simulink model "Model_InterpretationEngine64"  (R2022b)
settings: Solver=FixedStepDiscrete  StartTime=0.0  StopTime=5  RelTol=1e-3  EnableMultiTasking=on
InitFcn:
  | % Initialize model
  | ModelSettings=BTConfig.GetModelSettings();
  | 
  | ModelSettings.Validate();
  | 
  | ModelInit;
  | 
  | 
  | % load library data
  | GainLibrary_data;
  | % Load saved values from partition process
  | CapturedConstMask.LoadMapFromFile(bdroot)
  | % Load saved values from partition process
  | TSP_Mask.LoadMapFromFile(bdroot)
StartFcn:
  | % make sure all the simulated RTC requests are found
  | %RTC_SIM_OBJ.ValidateREQs();
undefined symbols (not defined in the file or in its folder): NumHFRefBPF, NumHFRefLPF
libraries: StateVar x112, TSP x56, FeaturePath x24
(part 1 of 5)
settings Model: Creator=kl13806  LastModifiedBy=mp55777
settings DataIOCC: ReturnWorkspaceOutputs=off
settings OptimizationCC: DefaultParameterBehavior=Inlined  DefaultUnderspecifiedDataType=single  EfficientTunableParamExpr=on
settings DebuggingCC: MergeDetectMultiDrivingBlocksExec=none  InheritedTsInSrcMsg=none  MultiTaskDSMMsg=none  ParameterPrecisionLossMsg=none  ParameterTunabilityLossMsg=error  UnconnectedInputMsg=warning  UnconnectedOutputMsg=warning  UnconnectedLineMsg=warning  UnknownTsInhSupMsg=none  SFUnexpectedBacktrackingDiag=warning  SFNoUnconditionalDefaultTransitionDiag=warning  SFExecutionAtInitializationDiag=none  SFMachineParentedDataDiag=warning
settings HardwareCC: ProdBitPerPointer=32  ProdBitPerSizeT=32  ProdBitPerPtrDiffT=32  ProdWordSize=32  ProdHWDeviceType=Intel->x86-32 (Windows32)  TargetBitPerPointer=64  TargetBitPerSizeT=64  TargetBitPerPtrDiffT=64  TargetLongLongMode=on  TargetIntDivRoundTo=Zero  TargetEndianess=LittleEndian  TargetWordSize=64  TargetHWDeviceType=MATLAB Host  ProdEqTarget=off
settings ModelReferenceCC: EnableRefExpFcnMdlSchedulingChecks=on  ModelReferenceNumInstancesAllowed=Single
settings SFSimCC: MATLABDynamicMemAlloc=off
settings RTWCC: Description=Embedded Coder (host-based shared library target)  SystemTargetFile=ert_shrlib.tlc  TLCOptions="-aTALARIA_ENGINE=\"Interpretation\""  TemplateMakefile=ert_default_tmf  RTWVerbose=off  RetainRTWFile=on  Toolchain=MinGW64 | gmake (64-bit Windows)  IncludeHyperlinkInReport=on
settings RTWCC: CustomHeaderCode=|
  | // Auto-generated code for model Model
  | /**** TSP TOKEN COMPATIBILITY HASH VALUES ****/
  | #define TSP_COMPAT {0xD202EF8DUL, 0xD716E441UL, 0xBB1AC2DBUL, 0x70247352UL, 0xD202EF8DUL}
  | #define TSP_COMPAT_NAME {"InputSelect", "PreAmp", "Near", "PostProcess", "TestRouter"}
  | #define TSP_COMPAT_NAME_HASH {0xF8044409UL, 0xC3A89EEBUL, 0xD67EB32FUL, 0x062DAD3BUL, 0x8CC5BE54UL}
  | /**** COMPAT HASH VALUES BY MODULE ****/
  | #define INPUTSELECT_TSP_COMPAT 0xD202EF8DUL
  | #define PREAMP_TSP_COMPAT 0xD716E441UL
  | #define NEAR_TSP_COMPAT 0xBB1AC2DBUL
  | #define POSTPROCESS_TSP_COMPAT 0x70247352UL
  | #define TESTROUTER_TSP_COMPAT 0xD202EF8DUL
  | /**** NAME HASH VALUES BY MODULE ****/
  | #define INPUTSELECT_TSP_NAME_HASH 0xF8044409UL
  | #define PREAMP_TSP_NAME_HASH 0xC3A89EEBUL
  | #define NEAR_TSP_NAME_HASH 0xD67EB32FUL
  | #define POSTPROCESS_TSP_NAME_HASH 0x062DAD3BUL
  | #define TESTROUTER_TSP_NAME_HASH 0x8CC5BE54UL
settings CodeAppCC: ForceParamTrailComments=on  IgnoreCustomStorageClasses=off  MaxIdLength=128  OperatorAnnotations=on  SimulinkDataObjDesc=on  SFDataObjDesc=on  MATLABFcnDesc=on  InsertBlockDesc=on  StateflowObjectComments=on  MATLABSourceComments=on
settings STFCustomTargetCC: TargetLangStandard=C99 (ISO)  MultiwordLength=256  ParMdlRefBuildCompliant=on  CompOptLevelCompliant=on  CombineOutputUpdateFcns=on  ERTCustomFileBanners=on  SupportContinuousTime=off  SupportNonInlinedSFcns=off  RemoveResetFunc=on  SupportVariableSizeSignals=on  MATLABClassNameForMDSCustomization=Simulink.SoftwareTarget.ERTCustomization  ModelStepFunctionPrototypeControlCompliant=on  UseToolchainInfoCompliant=on  SystemTargetFile=ert_shrlib.tlc
settings ERTTargetCC: TargetLangStandard=C99 (ISO)  ConcurrentExecutionCompliant=off  SupportVariableSizeSignals=on  CPPClassGenCompliant=off  InlinedParameterPlacement=NonHierarchical  ERTCustomFileTemplate=interpretation_dll.tlc  IndentStyle=Allman  IndentSize=4

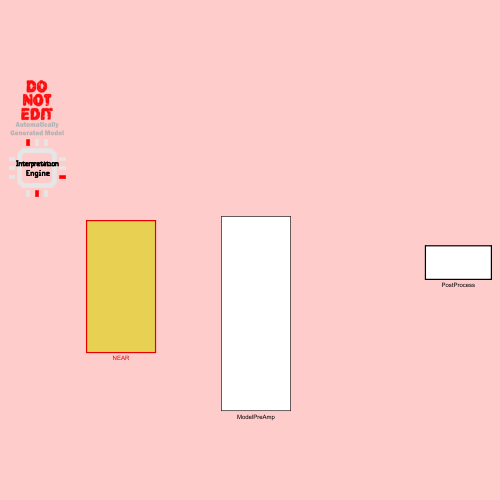
[thumbnail: Simulink's stored preview of the top-level diagram]
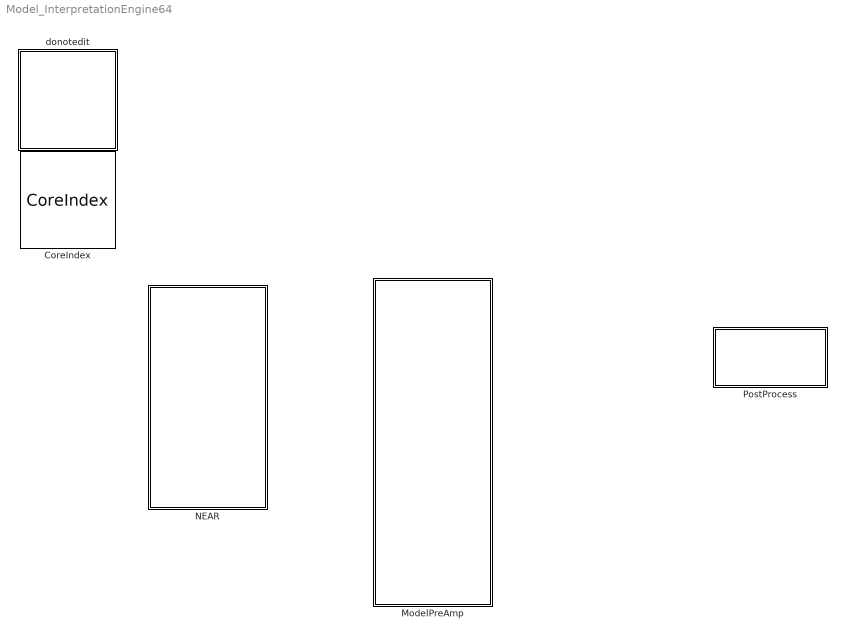
== system Model_InterpretationEngine64 ==
  CoreIndex : FeaturePath/CoreIndex  Role=Interpretation Engine  CoreIndex=10  Config=[]  AddressingMode=Indirect core determination via table lookup (i.e. use Partition blocks)  CrossCoreApi=None  CrossCoreAllocation=None  CrossCoreSampleTime=-1  BasePeriod=[]  TriggerInit=[440 234 535 331]
      settings: SourceProductName=Bose Talaria
  ModelPreAmp : Subsystem  mask{Config=ModelSettings.ModelPreAmp}
      mask prompts: Config "PreAmpConfig"
  NEAR : Subsystem  TreatAsAtomicUnit=on  mask{Config=ModelSettings.NearConfig}
      mask prompts: Config "NearConfig"
  PostProcess : Subsystem  TreatAsAtomicUnit=on  mask{Config=ModelSettings.PostProcess}
      mask prompts: Config "PostProcessConfig"
  donotedit : Subsystem
      settings: OpenFcn=Model
      mask Display: image('DoNotEdit.svg');

== system Model_InterpretationEngine64/ModelPreAmp ==
  DecRate : Subsystem
  FeaturePath : FeaturePath/FeaturePath  FeatureName=PreAmp  IsGroup=on  GroupNumber=2  IsModule=on  TriggerInit=[-135 -246 -20 -139]
      settings: SourceProductName=Bose Talaria

== system Model_InterpretationEngine64/NEAR ==
  FeaturePath : FeaturePath/FeaturePath  FeatureName=Near  IsGroup=on  GroupNumber=1  IsModule=on  TriggerInit=[15 -306 130 -199]
      settings: SourceProductName=Bose Talaria
  Near1p1 : Subsystem  mask{Config=Config.Near}
      mask prompts: Config "Near1p1Config"
      mask init:
      | blkh=gcbh;
      | Config=BTConfig.Assert(blkh,Config);
      | % sample_rate_in_hertz                        = near.sample_rate_in_hertz;
      | % frame_size                                  = near.frame_size;
      | % ann_sysin_channel_count                     = near.ann_sysin_channel_count;
      | % front_peripheral_channel_count              = near.front_peripheral_channel_count;
      | % NEAR1p1FrontPeripheralChannelCountFullRate  = near.NEAR1p1FrontPeripheralChannelCountFullRate;
      | % NearWbAnnCount                              = near.NearWbAnnCount;
      | % headrest_count                              = near.headrest_count;
      | % channels_per_headrest                       = near.channels_per_headrest;
      | % decimation_factor                           = near.decimation_factor;
      | % rear_channel_count                          = near.rear_channel_count;
      | % vm                                          = near.vm;
      | % decimated_frame_size                        = near.decimated_frame_size;
      | % decimated_sample_rate_in_hertz              = near.decimated_sample_rate_in_hertz;
      | Config.Validate();
      | Config.DoMaskInit(blkh);

== system Model_InterpretationEngine64/PostProcess ==
  FeaturePath : FeaturePath/FeaturePath  FeatureName=PostProcess  IsGroup=on  GroupNumber=3  IsModule=on  TriggerInit=[85 -186 200 -79]
      settings: SourceProductName=Bose Talaria
  PostProcess : Subsystem  TreatAsAtomicUnit=on
      settings: RTWSystemCode=Nonreusable function  RTWFcnNameOpts=Use subsystem name  RTWFileNameOpts=Use subsystem name  FunctionWithSeparateData=on

== system Model_InterpretationEngine64/donotedit ==

== system Model_InterpretationEngine64/ModelPreAmp/DecRate ==
  AudioPilot35 : Subsystem  TreatAsAtomicUnit=on
      settings: RTWFcnNameOpts=Use subsystem name  RTWFileNameOpts=Use subsystem name  FunctionWithSeparateData=on
  Medusa5H1 : Subsystem

== system Model_InterpretationEngine64/NEAR/Near1p1 ==
  VolumeMute : Subsystem  mask{Config=Config.VolumeMute}
      mask prompts: Config "VolumeMuteConfig"
      mask init:
      | blkh=gcbh;
      | Config=BTConfig.Assert(blkh,Config);
      | 
      | Config.Validate();
      | Config.DoMaskInit(blkh);

== system Model_InterpretationEngine64/PostProcess/PostProcess ==
  EnergyLimiter : Subsystem

== system Model_InterpretationEngine64/ModelPreAmp/DecRate/AudioPilot35 ==
  Audiopilot_3_5 : Subsystem  mask(AudioPilot 3.5){FeatureName=Audiopilot, InputAudioMode=Stereo - 2 Channels, NoiseEstimationMode=Regular, IncludeSpumTails=off, IncludeIgnoreMicFlag=off, Config=Config.Audiopilot}
      mask prompts: FeatureName "Feature Name:"; InputAudioMode "Input Audio Mode"; NoiseEstimationMode "Mode"; IncludeSpumTails "Include SPUM Tails as Reference Channels for High-Frequency Noise Estimator"; IncludeIgnoreMicFlag "Include Ignore Microphone Flag as Input"; Config "Audiopilot_3_5Config"
      mask help:
      | This is the top level model implementing AudioPilot 3.5.
      | It is configurable to accommodate both stereo inputs and surround inputs.  It can also reconfigure itself to become a speed-only implementation. For the regular implementation, there are two options. One is to allow a flag signal to instruct the algorithm to ignore the microphone signal; the other is to include in the set of "high-passed" reference channels the 2 channels representing the SPUM tails from the Medusa Upmixer.
      | Build Time Configuration settings typically set for this block include the frame size and the sample rate of the input audio. Other options include the type of code generation and whether all RTC blocks will generate a response.
      mask init:
      | blkh = gcbh;
      | 
      | Config = BTConfig.Assert(blkh,Config);
      | Config.Validate();
      | 
      | FrameSize = Config.FrameSize;
      | SampleRate = Config.SampleRateHz;
      |  
      | % Make the choice for the Noise Estimation Variant
      | Audiopilot_3_5Mask.ConfigureVariant(blkh,NoiseEstimationMode);
      | 
      | % Set up the number of audio channels for each input
      | [NumMicChannels,NumMusicChannels, ...
      |     NumHFRefLPF,NumHFRefBPF,NumLFRef] = ...
      |     Audiopilot_3_5Mask.ChannelSetUp(blkh,InputAudioMode,...
      |                 NoiseEstimationMode,IncludeSpumTails);
      | 
      | % Configure RTC responses            
      | Audiopilot_3_5Mask.ConfigureRtcResponses(blkh,...
      |                 Config.EnableRtcResponse)           
      | 
      | % Configure the Model according to Mask Parameters   
      | Audiopilot_3_5Mask.ConfigureModel(blkh,InputAudioMode,...
      |     NoiseEstimationMode,IncludeIgnoreMicFlag);
      | 
      | BTConfig.InitSetFeatureIfPresent(blkh,'FeatureName');
      mask TypeOptions FeatureName: FeaturePath/FeatureName
      mask TypeOptions InputAudioMode: Stereo - 2 Channels | Surround - 6 Channels
      mask TypeOptions NoiseEstimationMode: Regular | Speed Only
      mask Callback NoiseEstimationMode: Audiopilot_3_5Mask.NoiseEstimationModeCallBack(gcbh);
      mask Callback Config: BTConfig.CallbackHideIfPresent(gcbh,{'FeatureName'});
      mask DialogControl DTCTitle Prompt: <b> Design Time Configuration </b>
      mask DialogControl NoiseEstimationBox Prompt: Noise Estimation
      mask DialogControl BTCTitle Prompt: <b> Build Time Configuration </b>
  EntertainmentLevelDetection : Subsystem  mask(Level Detector for AudioPilot, Dyanmic EQ, Fan and Boost-on-Demand){NumInputChannels=Config.AudiopilotNumMusicIn, FANEnable=off, BODEnable=off, Config=Config.LDCfg}
      mask prompts: NumInputChannels "Number of Input Channels"; FANEnable "FAN (amplifier fan control)"; BODEnable "BOD (boost on demand)"; Config "EntertainmentLevelDetectionConfig"
      mask help: This block performs level detection, separately and independently, for various features. The features, AudioPilot and Dynamic Equalization, are always included. The other features, Amplifier Fan Control, and Boost on Demand, are optional. The block is designed to accept as input the entertainment audio channels before volume control was applied. The volume setting, in linear, forms a different input.
      mask init:
      | blkh = gcbh;
      | 
      | Config = BTConfig.Assert(blkh,Config);
      | Config.Validate();
      | 
      | SampleRate = Config.SampleRateHz;
      | FrameSize = Config.FrameSize;
      | FrameRate = Config.FrameRateHz;
      | MaxMusicDelay = Config.MaxMusicDelay;
      | MaxMusicDelayPerChannel = floor(MaxMusicDelay/NumInputChannels);
      | 
      | EntertainmentLevelDetectionMask.ConfigureAdditionalLevelDetectors ...
      |     (blkh,FANEnable,BODEnable)
      mask Help:
      | This block performs level detection for various features.
      | 
      | Arguments for this block:
      | 
      | Configuration
      | The block can be configured using a object of class, EntertainmentLevelDetectionConfig.  If the "use Default Configuration Only" box is checked, then this option is disabled.
      | 
      | Additional Level Estimates
      | FAN (amplifier fan control)
      | BOD (boost on demand)
      | 
      | System Definitions
      | Sample Rate --- Fs
      | Frame Size --- frameSize
      | Maximum Delay for the Music --- maxMusicDelay
      mask DialogControl DTC Prompt: Design Time Configuration
      mask DialogControl AdditionalGroup Prompt: Additional Level Estimates
      mask DialogControl BTC Prompt: Build Time Configuration

== system Model_InterpretationEngine64/ModelPreAmp/DecRate/Medusa5H1 ==
  MedusaHoligram : Subsystem  mask{config=Config.MedusaConfig, ConfigBTC=Config.MedusaBTC, vlsConfigStruct=Config.VLSConfig}
      mask prompts: config "Medusa config struct name:"; ConfigBTC "Medusa BTC config struct name:"; vlsConfigStruct "VLS config struct name:"
      mask init:
      | tailCompEQ = config.tailCompEQ;
      | HRDelayConfig = vlsConfigStruct.HeadrestDelayConfig;

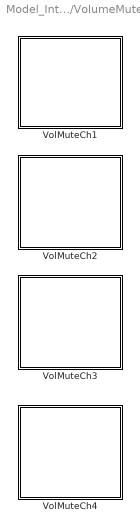
== system Model_InterpretationEngine64/NEAR/Near1p1/VolumeMute ==
  VolMuteCh1 : Subsystem
  VolMuteCh2 : Subsystem
  VolMuteCh3 : Subsystem
  VolMuteCh4 : Subsystem

== system Model_InterpretationEngine64/PostProcess/PostProcess/EnergyLimiter ==
  EnergyLimiter1 : Subsystem  mask(Blocklib EnergyLimiter){Config=Config.EnergyLimiter, FeatureName=EnergyLimiter}
      mask prompts: Config "EnergyLimiterConfig"; FeatureName "Feature path name:"
      mask help:
      | This block is used for reducing the gain of an audio signal based upon the crest factor of that signal. Such an algorithm is required for the new generations of amplifiers that have many output channels.
      |
      | Note:Please refer and click on Help tab to get details on configuration parameters
      mask init:
      | blkh=gcbh;
      | Config=BTConfig.Assert(blkh,Config);
      | 
      | Config.Validate();
      | BTConfig.InitSetFeatureIfPresent(blkh,'FeatureName');
      mask Help:
      | Configuration Parameters:
      | 
      |   GainChangeStepIndB
      |                         : Step in dB that gain should be changed by each time signal
      |                           crosses energy threshold. This number should be >= 0.
      | 
      |   GainIncreaseDurationInSeconds
      |                         : Duration that a gain increase should be applied before it
      |                           can be updated. This number should be > 0.
      | 
      |   GainDecreaseDurationInSeconds
      |                         : Duration that a gain decrease should be applied before it
      |                           can be updated. This number should be > 0.
      | 
      |   MaxEnergyLevelIndB
      |                         : Max energy level in dB for each channel above which gain
      |                           energy reduction should kick in. This number should be <= 0
      | 
      |   MaxChannels : Maximum number of channels that may be above energy level
      |                           threshold before gain reduction kicks in.
      |                           This number should be between 0 and numIn (inclusive).
      | 
      |   MaxGainReductionIndB
      |                         : Max gain reduction that should be done.
      |                           This number should be >= 0
      | 
      |   EnergyMeasurementTimeConstantInSeconds
      |                         : Time interval for averaging measured energy (in seconds).
      | 
      |   EnergyAdjustmentFactorIndB
      |                         : A Multiplier factor to adjust EBL threshold based on platform.
      |                           This number should be > 0.
      mask Callback Config: BTConfig.CallbackHideIfPresent(gcbh,{'FeatureName'});
      mask TypeOptions FeatureName: FeaturePath/FeatureName

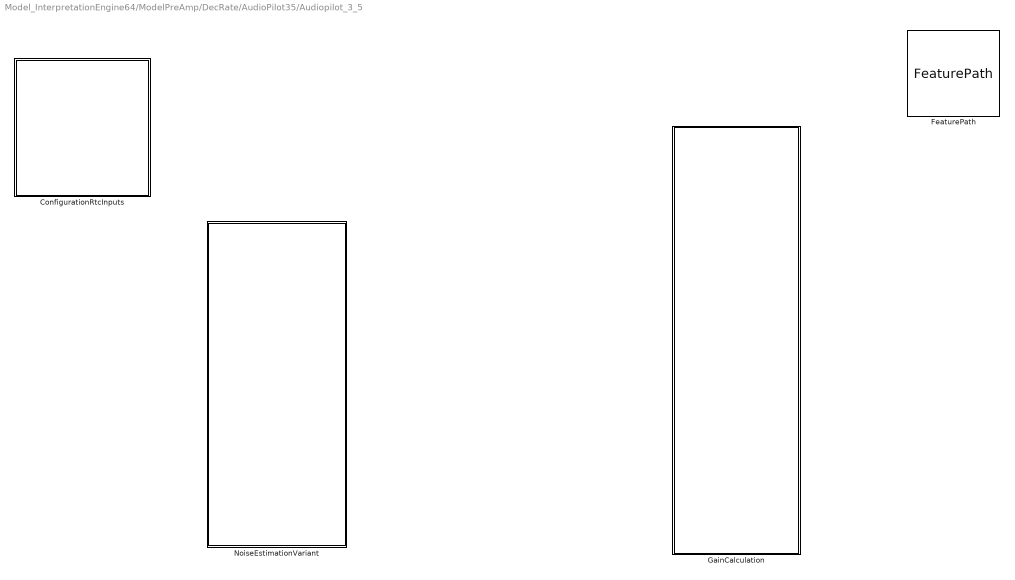
== system Model_InterpretationEngine64/ModelPreAmp/DecRate/AudioPilot35/Audiopilot_3_5 ==
  ConfigurationRtcInputs : Subsystem
  FeaturePath : FeaturePath/FeaturePath  FeatureName=Audiopilot  IsGroup=off  GroupNumber=-1  IsModule=off  TriggerInit=[1175 264 1290 371]
      settings: SourceProductName=Bose Talaria
  GainCalculation : Subsystem  mask(AudioPilot - Gain Calculation){Config=Config.GainCalc}
      mask prompts: Config "GainCalculationConfig"
      mask help: This block implements the gain calculations for AudioPilot and Dynamic EQ.
      mask init:
      | blkh = gcbh;
      | 
      | Config = BTConfig.Assert(blkh,Config);
      | Config.Validate();
      | 
      | SampleRate = Config.SampleRateHz;
      | FrameSize = Config.FrameSize;
      | FrameRate = Config.FrameRateHz;
      | 
      | % Configure RTC responses            
      | GainCalculationMask.ConfigureRtcResponses(blkh,...
      |                 Config.EnableRtcResponse)
      mask Help:
      | This block implements the gain calculations for AudioPilot and Dynamic EQ.
      | 
      | Arguments for this block:
      | 
      | Configuration
      | The block can be configured using an object of class, GainCalculationConfig.
      mask DialogControl BTC Prompt: Build Time Configuration
      mask DialogControl Config Tooltip: The configuration has to be an object of the class, GainCalculationConfig.
  NoiseEstimationVariant : Subsystem  Variant=on  VariantControlMode=label  LabelModeActiveChoice=Regular  PropagateVariantConditions=on

== system Model_InterpretationEngine64/ModelPreAmp/DecRate/AudioPilot35/EntertainmentLevelDetection ==
  AudiopilotLevelDetect : Subsystem
  DyneqLevelDetect : Subsystem

== system Model_InterpretationEngine64/ModelPreAmp/DecRate/Medusa5H1/MedusaHoligram ==
  FeaturePath : FeaturePath/FeaturePath  FeatureName=Medusa  IsGroup=off  GroupNumber=-1  IsModule=off  TriggerInit=[90 69 205 176]
      settings: SourceProductName=Bose Talaria
  Medusa5H1 Part 1 : Subsystem  TreatAsAtomicUnit=on
      settings: RTWSystemCode=Nonreusable function
  Medusa5H1 Part 2 : Subsystem  TreatAsAtomicUnit=on
      settings: RTWSystemCode=Nonreusable function

== system Model_InterpretationEngine64/NEAR/Near1p1/VolumeMute/VolMuteCh1 ==
  Ann1NonEntGainCalc : Subsystem  mask(Blocklib NonEntGainCalc){Config=Config.Ann1NonEntGainCalc, FeatureName=Ann1NonEntGainCalc}
      mask prompts: Config "NonEntGainCalcConfig"; FeatureName "Feature path name:"
      mask init:
      | blkh=gcbh;
      | Config=BTConfig.Assert(blkh,Config);
      | 
      | Config.Validate();
      | BTConfig.InitSetFeatureIfPresent(blkh,'FeatureName');
      | 
      | % Flatten for MFB is not needed due to mask on MFB. Nice.
      mask Callback Config: BTConfig.CallbackHideIfPresent(gcbh,{'FeatureName'});
      mask TypeOptions FeatureName: FeaturePath/FeatureName
      mask DialogControl ParameterGroupVar2 Prompt: OverRides
  FeaturePath : FeaturePath/FeaturePath  FeatureName=Ann1  IsGroup=off  GroupNumber=-1  IsModule=off  TriggerInit=[270 -291 385 -184]
      settings: SourceProductName=Bose Talaria

== system Model_InterpretationEngine64/NEAR/Near1p1/VolumeMute/VolMuteCh2 ==
  Ann2NonEntGainCalc : Subsystem  mask(Blocklib NonEntGainCalc){Config=Config.Ann2NonEntGainCalc, FeatureName=Ann2NonEntGainCalc}
      mask prompts: Config "NonEntGainCalcConfig"; FeatureName "Feature path name:"
      mask init:
      | blkh=gcbh;
      | Config=BTConfig.Assert(blkh,Config);
      | 
      | Config.Validate();
      | BTConfig.InitSetFeatureIfPresent(blkh,'FeatureName');
      | 
      | % Flatten for MFB is not needed due to mask on MFB. Nice.
      mask Callback Config: BTConfig.CallbackHideIfPresent(gcbh,{'FeatureName'});
      mask TypeOptions FeatureName: FeaturePath/FeatureName
      mask DialogControl ParameterGroupVar2 Prompt: OverRides
  FeaturePath : FeaturePath/FeaturePath  FeatureName=Ann2  IsGroup=off  GroupNumber=-1  IsModule=off  TriggerInit=[60 -206 175 -99]
      settings: SourceProductName=Bose Talaria

== system Model_InterpretationEngine64/NEAR/Near1p1/VolumeMute/VolMuteCh3 ==
  Ann3NonEntGainCalc : Subsystem  mask(Blocklib NonEntGainCalc){Config=Config.Ann3NonEntGainCalc, FeatureName=Ann3NonEntGainCalc}
      mask prompts: Config "NonEntGainCalcConfig"; FeatureName "Feature path name:"
      mask init:
      | blkh=gcbh;
      | Config=BTConfig.Assert(blkh,Config);
      | 
      | Config.Validate();
      | BTConfig.InitSetFeatureIfPresent(blkh,'FeatureName');
      | 
      | % Flatten for MFB is not needed due to mask on MFB. Nice.
      mask Callback Config: BTConfig.CallbackHideIfPresent(gcbh,{'FeatureName'});
      mask TypeOptions FeatureName: FeaturePath/FeatureName
      mask DialogControl ParameterGroupVar2 Prompt: OverRides
  FeaturePath : FeaturePath/FeaturePath  FeatureName=Ann3  IsGroup=off  GroupNumber=-1  IsModule=off  TriggerInit=[265 -336 380 -229]
      settings: SourceProductName=Bose Talaria

== system Model_InterpretationEngine64/NEAR/Near1p1/VolumeMute/VolMuteCh4 ==
  Ann4NonEntGainCalc : Subsystem  mask(Blocklib NonEntGainCalc){Config=Config.Ann4NonEntGainCalc, FeatureName=Ann4NonEntGainCalc}
      mask prompts: Config "NonEntGainCalcConfig"; FeatureName "Feature path name:"
      mask init:
      | blkh=gcbh;
      | Config=BTConfig.Assert(blkh,Config);
      | 
      | Config.Validate();
      | BTConfig.InitSetFeatureIfPresent(blkh,'FeatureName');
      | 
      | % Flatten for MFB is not needed due to mask on MFB. Nice.
      mask Callback Config: BTConfig.CallbackHideIfPresent(gcbh,{'FeatureName'});
      mask TypeOptions FeatureName: FeaturePath/FeatureName
      mask DialogControl ParameterGroupVar2 Prompt: OverRides
  FeaturePath : FeaturePath/FeaturePath  FeatureName=Ann4  IsGroup=off  GroupNumber=-1  IsModule=off  TriggerInit=[235 -186 350 -79]
      settings: SourceProductName=Bose Talaria

== system Model_InterpretationEngine64/PostProcess/PostProcess/EnergyLimiter/EnergyLimiter1 ==
  note: The algorithm maintains a moving average of the energy of the input signal as follows:
      | AverageEnergy[n] Energy[n] + AverageEnergy[n-1]
      | where Energy[n] is the energy for frame n and is an averaging constant.
  "EnergyRunningAvg " : Subsystem
  FeaturePath : FeaturePath/FeaturePath  FeatureName=EnergyLimiter  IsGroup=off  GroupNumber=-1  IsModule=off  TriggerInit=[680 174 795 281]
      settings: SourceProductName=Bose Talaria

== system Model_InterpretationEngine64/ModelPreAmp/DecRate/AudioPilot35/Audiopilot_3_5/ConfigurationRtcInputs ==
  note: Downgrade Flag
  note: HVAC
  note: Speed
  note: Mute
  APHvac : Subsystem  mask(Talaria Target State Variable){TriggerInit=[1390 1281 1530 1349], TspName=HvacDbspl, StateName=HvacDbspl, UseSameName=on, IfdefMacro=[]}
      mask prompts: TriggerInit "Hidden: MoveFcn redraw"; TspName "Name:"; StateName "Name of StateVar:"; UseSameName "Use same name for state variable and TSP"; IfdefMacro "Additional #ifdef macro to enable trigger capture:"
      mask help: The TargetStateVar block encapsultes a Target State Probe (TSP), a State Variable, and a Trivial Interpretation between them.
      mask init:
      | [ok,tspPath,activeStatePath] = TargetStateVarMask.Init(gcbh);
      settings: MoveFcn=TargetStateVarMask.CB_TriggerInit(gcbh);
      mask Help: See help for StateVar and TSP blocks
      mask Callback TriggerInit: TargetStateVarMask.CB_TriggerInit(gcbh);
      mask TypeOptions TspName: TSP/TspName
      mask TypeOptions StateName: StateVar/StateName
      mask Callback UseSameName: TargetStateVarMask.CB_UseSameName(gcbh);
      mask TypeOptions IfdefMacro: TSP/IfdefMacro
      mask DialogControl AdvancedPanel Prompt: Advanced
      mask DialogControl ConvertToFullInterpretation Prompt: Irreversible conversion to full interpretation
      mask DialogControl ConvertToFullInterpretation Callback: TargetStateVarMask.CB_ConvertToFullInterpretation(gcbh);
      mask DialogControl ErrorContainer Prompt: Error Messages
      mask DialogControl ErrorText Prompt: The interpreted StateVar value is not yet available
      mask DialogControl TspPathText Prompt: TSP: Current parameter name: [AudiopilotHvacDbspl]
      mask Display:
      | % retrieve icon definition
      | [path,w,h] = TargetStateVarMask.Icon();
      | 
      | % retrieve the block's pixel size
      | pos = get(gcbh,'position');
      | bw = pos(3) - pos(1);
      | bh = pos(4) - pos(2);
      | 
      | % draw centered icon
      | xAdj = bw/2 - w/2 + 5;
      | yAdj = bh/2 - h/2 + 4;
      | for i=1:length(path)
      | 	patch(path(i).x+xAdj, path(i).y+yAdj, path(i).rgb);
      | end
      | 
      | % show the top name or an X
      | if (exist('ok','var') && ok)
      | 	text(bw*0.5, bh*0.2, tspPath, 'horizontalAlignment', 'center');
      | 	patch(0,0,[1 1 1]);
      | 	patch(bw,bh,[1 1 1]);
      | else
      | 	tx=bw*0.03;
      | 	ty=bh*0.03;
      | 	patch([0 tx bw bw-tx], [ty 0 bh-ty bh], [1 0 0]);
      | 	patch([0 bw-tx bw tx], [bh-ty 0 ty bh], [1 0 0]);
      | end
  VehicleSpeed : Subsystem  mask(Talaria Target State Variable){TriggerInit=[1345 1086 1485 1154], TspName=VehicleSpeed, StateName=VehicleSpeed, UseSameName=on, IfdefMacro=[]}
      mask prompts: TriggerInit "Hidden: MoveFcn redraw"; TspName "Name:"; StateName "Name of StateVar:"; UseSameName "Use same name for state variable and TSP"; IfdefMacro "Additional #ifdef macro to enable trigger capture:"
      mask help: The TargetStateVar block encapsultes a Target State Probe (TSP), a State Variable, and a Trivial Interpretation between them.
      mask init:
      | [ok,tspPath,activeStatePath] = TargetStateVarMask.Init(gcbh);
      settings: MoveFcn=TargetStateVarMask.CB_TriggerInit(gcbh);
      mask Help: See help for StateVar and TSP blocks
      mask Callback TriggerInit: TargetStateVarMask.CB_TriggerInit(gcbh);
      mask TypeOptions TspName: TSP/TspName
      mask TypeOptions StateName: StateVar/StateName
      mask Callback UseSameName: TargetStateVarMask.CB_UseSameName(gcbh);
      mask TypeOptions IfdefMacro: TSP/IfdefMacro
      mask DialogControl AdvancedPanel Prompt: Advanced
      mask DialogControl ConvertToFullInterpretation Prompt: Irreversible conversion to full interpretation
      mask DialogControl ConvertToFullInterpretation Callback: TargetStateVarMask.CB_ConvertToFullInterpretation(gcbh);
      mask DialogControl ErrorContainer Prompt: Error Messages
      mask DialogControl ErrorText Prompt: The interpreted StateVar value is not yet available
      mask DialogControl TspPathText Prompt: TSP: Current parameter name: [AudiopilotVehicleSpeed]
      mask Display:
      | % retrieve icon definition
      | [path,w,h] = TargetStateVarMask.Icon();
      | 
      | % retrieve the block's pixel size
      | pos = get(gcbh,'position');
      | bw = pos(3) - pos(1);
      | bh = pos(4) - pos(2);
      | 
      | % draw centered icon
      | xAdj = bw/2 - w/2 + 5;
      | yAdj = bh/2 - h/2 + 4;
      | for i=1:length(path)
      | 	patch(path(i).x+xAdj, path(i).y+yAdj, path(i).rgb);
      | end
      | 
      | % show the top name or an X
      | if (exist('ok','var') && ok)
      | 	text(bw*0.5, bh*0.2, tspPath, 'horizontalAlignment', 'center');
      | 	patch(0,0,[1 1 1]);
      | 	patch(bw,bh,[1 1 1]);
      | else
      | 	tx=bw*0.03;
      | 	ty=bh*0.03;
      | 	patch([0 tx bw bw-tx], [ty 0 bh-ty bh], [1 0 0]);
      | 	patch([0 bw-tx bw tx], [bh-ty 0 ty bh], [1 0 0]);
      | end

== system Model_InterpretationEngine64/ModelPreAmp/DecRate/AudioPilot35/Audiopilot_3_5/GainCalculation ==
  note: Gain Calculation
  Monitoring : Subsystem
  RampedEnable : Subsystem

== system Model_InterpretationEngine64/ModelPreAmp/DecRate/AudioPilot35/Audiopilot_3_5/NoiseEstimationVariant ==
  RegularNoiseEstimation : Subsystem  VariantControl=Regular
  SpeedOnly : Subsystem  VariantControl=Speed Only  mask(AudioPilot - Speed Only Noise Estimation){Config=Config.SpeedOnly}
      mask prompts: Config "SpeedOnlyConfig"
      mask help: This block implements the speed only variant for noise estimation
      mask init:
      | blkh = gcbh;
      | 
      | Config = BTConfig.Assert(blkh,Config);
      | Config.Validate();
      | 
      | SampleRate = Config.SampleRateHz;
      | DecRate = Config.DecRateHz;
      mask Help:
      | This block implements the speed only variant for noise estimation.
      | 
      | Arguments for this block:
      | 
      | Configuration
      | The block can be configured using an object of class, SpeedOnlyConfig.  If the "use Default Configuration Only" box is checked, then this option is disabled.
      | 
      | Sample Rate
      | This is the sample rate of the input audio streams, typically 44100 Hz or 48 kHz.
      mask DialogControl BTC Prompt: Build Time Configuration
      mask DialogControl Config Tooltip: The configuration has to be an object of the class, SpeedOnlyConfig.

== system Model_InterpretationEngine64/ModelPreAmp/DecRate/AudioPilot35/EntertainmentLevelDetection/AudiopilotLevelDetect ==
  Monitor : Subsystem

== system Model_InterpretationEngine64/ModelPreAmp/DecRate/AudioPilot35/EntertainmentLevelDetection/DyneqLevelDetect ==
  Monitor : Subsystem

== system Model_InterpretationEngine64/ModelPreAmp/DecRate/Medusa5H1/MedusaHoligram/Medusa5H1 Part 1 ==
  CAE Treble Boost : Subsystem  Variant=on

== system Model_InterpretationEngine64/ModelPreAmp/DecRate/Medusa5H1/MedusaHoligram/Medusa5H1 Part 2 ==
  Mono Detector : Subsystem  mask(Mono Detector){Config=ConfigBTC.MonoDetector}
      mask prompts: Config "MedusaMonoDetectorConfig"
      mask help:
      | This block detects if given stereo input (L, R) is stereo. The output isStereo is used to enable/disable Spatial Unmasker in Medusa system. When the block is put to passthrough by tuning, the default output is set to 'true'.
      |
      | Configuration struct needs to define the below fields with the exact names which are used inside the block.
      |
      | decimationFactor: decimation factor
      | maxZeroLevelCount: maximum number of zero signals in a row before reset
      | hpfOrder: order of highpass filter
      | maxNumStages: maximum of sos for both L and R highpass filter
      | numChannels: number of channels
      |
      | For more information and sample generation of config struct, please see 'Help'.
      mask init:
      | blkh=gcbh;
      | Config=BTConfig.Assert(blkh,Config);
      | 
      | Config.Validate();
      mask Help:
      | Model that uses Mono Detector block need to call MonoDetectorInit(config) to generate <i>MonoDetectorConfigStruct</i> and <i>MonoDetectorTunable</i> bus object in base workspace.
      | 
      | <b>Sample usage:</b>
      | 
      | MedusaConfig = generateMedusaConfig(auto_gen_sys_defs);
      | MonoDetectorInit(MedusaConfig);
      | or
      | DefaultMedusaConfig = generateMedusaConfig();
      | MonoDetectorInit(DefaultMedusaConfig);

== system Model_InterpretationEngine64/NEAR/Near1p1/VolumeMute/VolMuteCh1/Ann1NonEntGainCalc ==
  FeaturePath : FeaturePath/FeaturePath  FeatureName=Ann1NonEntGainCalc  IsGroup=off  GroupNumber=-1  IsModule=off  TriggerInit=[-350 -126 -235 -19]
      settings: SourceProductName=Bose Talaria
  boost : Subsystem

== system Model_InterpretationEngine64/NEAR/Near1p1/VolumeMute/VolMuteCh2/Ann2NonEntGainCalc ==
  FeaturePath : FeaturePath/FeaturePath  FeatureName=Ann2NonEntGainCalc  IsGroup=off  GroupNumber=-1  IsModule=off  TriggerInit=[-350 -126 -235 -19]
      settings: SourceProductName=Bose Talaria
  boost : Subsystem

== system Model_InterpretationEngine64/NEAR/Near1p1/VolumeMute/VolMuteCh3/Ann3NonEntGainCalc ==
  FeaturePath : FeaturePath/FeaturePath  FeatureName=Ann3NonEntGainCalc  IsGroup=off  GroupNumber=-1  IsModule=off  TriggerInit=[-350 -126 -235 -19]
      settings: SourceProductName=Bose Talaria
  boost : Subsystem

== system Model_InterpretationEngine64/NEAR/Near1p1/VolumeMute/VolMuteCh4/Ann4NonEntGainCalc ==
  FeaturePath : FeaturePath/FeaturePath  FeatureName=Ann4NonEntGainCalc  IsGroup=off  GroupNumber=-1  IsModule=off  TriggerInit=[-350 -126 -235 -19]
      settings: SourceProductName=Bose Talaria
  boost : Subsystem

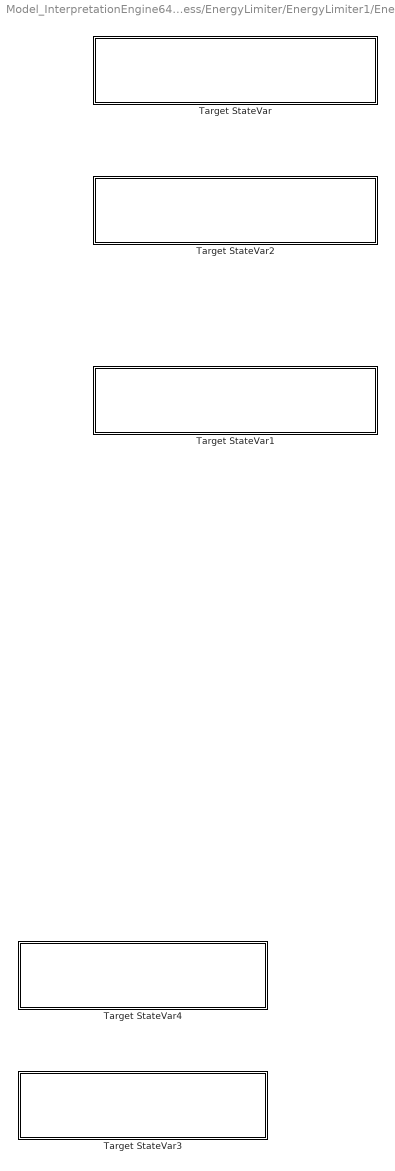
== system Model_InterpretationEngine64/PostProcess/PostProcess/EnergyLimiter/EnergyLimiter1/EnergyRunningAvg  ==
  Target StateVar : Subsystem  mask(Talaria Target State Variable){TriggerInit=[1755 218 2035 282], TspName=ComputedEnergy, StateName=ComputedEnergy, UseSameName=on, IfdefMacro=[]}
      mask prompts: TriggerInit "Hidden: MoveFcn redraw"; TspName "Name:"; StateName "Name of StateVar:"; UseSameName "Use same name for state variable and TSP"; IfdefMacro "Additional #ifdef macro to enable trigger capture:"
      mask help: The TargetStateVar block encapsultes a Target State Probe (TSP), a State Variable, and a Trivial Interpretation between them.
      mask init:
      | [ok,tspPath,activeStatePath] = TargetStateVarMask.Init(gcbh);
      settings: MoveFcn=TargetStateVarMask.CB_TriggerInit(gcbh);
      mask Help: See help for StateVar and TSP blocks
      mask Callback TriggerInit: TargetStateVarMask.CB_TriggerInit(gcbh);
      mask TypeOptions TspName: TSP/TspName
      mask TypeOptions StateName: StateVar/StateName
      mask Callback UseSameName: TargetStateVarMask.CB_UseSameName(gcbh);
      mask TypeOptions IfdefMacro: TSP/IfdefMacro
      mask DialogControl AdvancedPanel Prompt: Advanced
      mask DialogControl ConvertToFullInterpretation Prompt: Irreversible conversion to full interpretation
      mask DialogControl ConvertToFullInterpretation Callback: TargetStateVarMask.CB_ConvertToFullInterpretation(gcbh);
      mask DialogControl ErrorContainer Prompt: Error Messages
      mask DialogControl ErrorText Prompt: The interpreted StateVar value is not yet available
      mask DialogControl TspPathText Prompt: TSP: Current parameter name: [PostProcessEnergyLimiterComputedEnergy]
      mask Display:
      | % retrieve icon definition
      | [path,w,h] = TargetStateVarMask.Icon();
      | 
      | % retrieve the block's pixel size
      | pos = get(gcbh,'position');
      | bw = pos(3) - pos(1);
      | bh = pos(4) - pos(2);
      | 
      | % draw centered icon
      | xAdj = bw/2 - w/2 + 5;
      | yAdj = bh/2 - h/2 + 4;
      | for i=1:length(path)
      | 	patch(path(i).x+xAdj, path(i).y+yAdj, path(i).rgb);
      | end
      | 
      | % show the top name or an X
      | if (exist('ok','var') && ok)
      | 	text(bw*0.5, bh*0.2, tspPath, 'horizontalAlignment', 'center');
      | 	patch(0,0,[1 1 1]);
      | 	patch(bw,bh,[1 1 1]);
      | else
      | 	tx=bw*0.03;
      | 	ty=bh*0.03;
      | 	patch([0 tx bw bw-tx], [ty 0 bh-ty bh], [1 0 0]);
      | 	patch([0 bw-tx bw tx], [bh-ty 0 ty bh], [1 0 0]);
      | end
  Target StateVar1 : Subsystem  mask(Talaria Target State Variable){TriggerInit=[1755 548 2035 612], TspName=CurGain, StateName=CurGain, UseSameName=on, IfdefMacro=[]}
      mask prompts: TriggerInit "Hidden: MoveFcn redraw"; TspName "Name:"; StateName "Name of StateVar:"; UseSameName "Use same name for state variable and TSP"; IfdefMacro "Additional #ifdef macro to enable trigger capture:"
      mask help: The TargetStateVar block encapsultes a Target State Probe (TSP), a State Variable, and a Trivial Interpretation between them.
      mask init:
      | [ok,tspPath,activeStatePath] = TargetStateVarMask.Init(gcbh);
      settings: MoveFcn=TargetStateVarMask.CB_TriggerInit(gcbh);
      mask Help: See help for StateVar and TSP blocks
      mask Callback TriggerInit: TargetStateVarMask.CB_TriggerInit(gcbh);
      mask TypeOptions TspName: TSP/TspName
      mask TypeOptions StateName: StateVar/StateName
      mask Callback UseSameName: TargetStateVarMask.CB_UseSameName(gcbh);
      mask TypeOptions IfdefMacro: TSP/IfdefMacro
      mask DialogControl AdvancedPanel Prompt: Advanced
      mask DialogControl ConvertToFullInterpretation Prompt: Irreversible conversion to full interpretation
      mask DialogControl ConvertToFullInterpretation Callback: TargetStateVarMask.CB_ConvertToFullInterpretation(gcbh);
      mask DialogControl ErrorContainer Prompt: Error Messages
      mask DialogControl ErrorText Prompt: The interpreted StateVar value is not yet available
      mask DialogControl TspPathText Prompt: TSP: Current parameter name: [PostProcessEnergyLimiterCurGain]
      mask Display:
      | % retrieve icon definition
      | [path,w,h] = TargetStateVarMask.Icon();
      | 
      | % retrieve the block's pixel size
      | pos = get(gcbh,'position');
      | bw = pos(3) - pos(1);
      | bh = pos(4) - pos(2);
      | 
      | % draw centered icon
      | xAdj = bw/2 - w/2 + 5;
      | yAdj = bh/2 - h/2 + 4;
      | for i=1:length(path)
      | 	patch(path(i).x+xAdj, path(i).y+yAdj, path(i).rgb);
      | end
      | 
      | % show the top name or an X
      | if (exist('ok','var') && ok)
      | 	text(bw*0.5, bh*0.2, tspPath, 'horizontalAlignment', 'center');
      | 	patch(0,0,[1 1 1]);
      | 	patch(bw,bh,[1 1 1]);
      | else
      | 	tx=bw*0.03;
      | 	ty=bh*0.03;
      | 	patch([0 tx bw bw-tx], [ty 0 bh-ty bh], [1 0 0]);
      | 	patch([0 bw-tx bw tx], [bh-ty 0 ty bh], [1 0 0]);
      | end
  Target StateVar2 : Subsystem  mask(Talaria Target State Variable){TriggerInit=[1755 358 2035 422], TspName=EnergyThreshold, StateName=EnergyThreshold, UseSameName=on, IfdefMacro=[]}
      mask prompts: TriggerInit "Hidden: MoveFcn redraw"; TspName "Name:"; StateName "Name of StateVar:"; UseSameName "Use same name for state variable and TSP"; IfdefMacro "Additional #ifdef macro to enable trigger capture:"
      mask help: The TargetStateVar block encapsultes a Target State Probe (TSP), a State Variable, and a Trivial Interpretation between them.
      mask init:
      | [ok,tspPath,activeStatePath] = TargetStateVarMask.Init(gcbh);
      settings: MoveFcn=TargetStateVarMask.CB_TriggerInit(gcbh);
      mask Help: See help for StateVar and TSP blocks
      mask Callback TriggerInit: TargetStateVarMask.CB_TriggerInit(gcbh);
      mask TypeOptions TspName: TSP/TspName
      mask TypeOptions StateName: StateVar/StateName
      mask Callback UseSameName: TargetStateVarMask.CB_UseSameName(gcbh);
      mask TypeOptions IfdefMacro: TSP/IfdefMacro
      mask DialogControl AdvancedPanel Prompt: Advanced
      mask DialogControl ConvertToFullInterpretation Prompt: Irreversible conversion to full interpretation
      mask DialogControl ConvertToFullInterpretation Callback: TargetStateVarMask.CB_ConvertToFullInterpretation(gcbh);
      mask DialogControl ErrorContainer Prompt: Error Messages
      mask DialogControl ErrorText Prompt: The interpreted StateVar value is not yet available
      mask DialogControl TspPathText Prompt: TSP: Current parameter name: [PostProcessEnergyLimiterEnergyThreshold]
      mask Display:
      | % retrieve icon definition
      | [path,w,h] = TargetStateVarMask.Icon();
      | 
      | % retrieve the block's pixel size
      | pos = get(gcbh,'position');
      | bw = pos(3) - pos(1);
      | bh = pos(4) - pos(2);
      | 
      | % draw centered icon
      | xAdj = bw/2 - w/2 + 5;
      | yAdj = bh/2 - h/2 + 4;
      | for i=1:length(path)
      | 	patch(path(i).x+xAdj, path(i).y+yAdj, path(i).rgb);
      | end
      | 
      | % show the top name or an X
      | if (exist('ok','var') && ok)
      | 	text(bw*0.5, bh*0.2, tspPath, 'horizontalAlignment', 'center');
      | 	patch(0,0,[1 1 1]);
      | 	patch(bw,bh,[1 1 1]);
      | else
      | 	tx=bw*0.03;
      | 	ty=bh*0.03;
      | 	patch([0 tx bw bw-tx], [ty 0 bh-ty bh], [1 0 0]);
      | 	patch([0 bw-tx bw tx], [bh-ty 0 ty bh], [1 0 0]);
      | end
  Target StateVar3 : Subsystem  mask(Talaria Target State Variable){TriggerInit=[1680 1253 1925 1317], TspName=CurState, StateName=CurState, UseSameName=on, IfdefMacro=[]}
      mask prompts: TriggerInit "Hidden: MoveFcn redraw"; TspName "Name:"; StateName "Name of StateVar:"; UseSameName "Use same name for state variable and TSP"; IfdefMacro "Additional #ifdef macro to enable trigger capture:"
      mask help: The TargetStateVar block encapsultes a Target State Probe (TSP), a State Variable, and a Trivial Interpretation between them.
      mask init:
      | [ok,tspPath,activeStatePath] = TargetStateVarMask.Init(gcbh);
      settings: MoveFcn=TargetStateVarMask.CB_TriggerInit(gcbh);
      mask Help: See help for StateVar and TSP blocks
      mask Callback TriggerInit: TargetStateVarMask.CB_TriggerInit(gcbh);
      mask TypeOptions TspName: TSP/TspName
      mask TypeOptions StateName: StateVar/StateName
      mask Callback UseSameName: TargetStateVarMask.CB_UseSameName(gcbh);
      mask TypeOptions IfdefMacro: TSP/IfdefMacro
      mask DialogControl AdvancedPanel Prompt: Advanced
      mask DialogControl ConvertToFullInterpretation Prompt: Irreversible conversion to full interpretation
      mask DialogControl ConvertToFullInterpretation Callback: TargetStateVarMask.CB_ConvertToFullInterpretation(gcbh);
      mask DialogControl ErrorContainer Prompt: Error Messages
      mask DialogControl ErrorText Prompt: The interpreted StateVar value is not yet available
      mask DialogControl TspPathText Prompt: TSP: Current parameter name: [PostProcessEnergyLimiterCurState]
      mask Display:
      | % retrieve icon definition
      | [path,w,h] = TargetStateVarMask.Icon();
      | 
      | % retrieve the block's pixel size
      | pos = get(gcbh,'position');
      | bw = pos(3) - pos(1);
      | bh = pos(4) - pos(2);
      | 
      | % draw centered icon
      | xAdj = bw/2 - w/2 + 5;
      | yAdj = bh/2 - h/2 + 4;
      | for i=1:length(path)
      | 	patch(path(i).x+xAdj, path(i).y+yAdj, path(i).rgb);
      | end
      | 
      | % show the top name or an X
      | if (exist('ok','var') && ok)
      | 	text(bw*0.5, bh*0.2, tspPath, 'horizontalAlignment', 'center');
      | 	patch(0,0,[1 1 1]);
      | 	patch(bw,bh,[1 1 1]);
      | else
      | 	tx=bw*0.03;
      | 	ty=bh*0.03;
      | 	patch([0 tx bw bw-tx], [ty 0 bh-ty bh], [1 0 0]);
      | 	patch([0 bw-tx bw tx], [bh-ty 0 ty bh], [1 0 0]);
      | end
  Target StateVar4 : Subsystem  mask(Talaria Target State Variable){TriggerInit=[1680 1123 1925 1187], TspName=EnableFlag, StateName=EnableFlag, UseSameName=on, IfdefMacro=[]}
      mask prompts: TriggerInit "Hidden: MoveFcn redraw"; TspName "Name:"; StateName "Name of StateVar:"; UseSameName "Use same name for state variable and TSP"; IfdefMacro "Additional #ifdef macro to enable trigger capture:"
      mask help: The TargetStateVar block encapsultes a Target State Probe (TSP), a State Variable, and a Trivial Interpretation between them.
      mask init:
      | [ok,tspPath,activeStatePath] = TargetStateVarMask.Init(gcbh);
      settings: MoveFcn=TargetStateVarMask.CB_TriggerInit(gcbh);
      mask Help: See help for StateVar and TSP blocks
      mask Callback TriggerInit: TargetStateVarMask.CB_TriggerInit(gcbh);
      mask TypeOptions TspName: TSP/TspName
      mask TypeOptions StateName: StateVar/StateName
      mask Callback UseSameName: TargetStateVarMask.CB_UseSameName(gcbh);
      mask TypeOptions IfdefMacro: TSP/IfdefMacro
      mask DialogControl AdvancedPanel Prompt: Advanced
      mask DialogControl ConvertToFullInterpretation Prompt: Irreversible conversion to full interpretation
      mask DialogControl ConvertToFullInterpretation Callback: TargetStateVarMask.CB_ConvertToFullInterpretation(gcbh);
      mask DialogControl ErrorContainer Prompt: Error Messages
      mask DialogControl ErrorText Prompt: The interpreted StateVar value is not yet available
      mask DialogControl TspPathText Prompt: TSP: Current parameter name: [PostProcessEnergyLimiterEnableFlag]
      mask Display:
      | % retrieve icon definition
      | [path,w,h] = TargetStateVarMask.Icon();
      | 
      | % retrieve the block's pixel size
      | pos = get(gcbh,'position');
      | bw = pos(3) - pos(1);
      | bh = pos(4) - pos(2);
      | 
      | % draw centered icon
      | xAdj = bw/2 - w/2 + 5;
      | yAdj = bh/2 - h/2 + 4;
      | for i=1:length(path)
      | 	patch(path(i).x+xAdj, path(i).y+yAdj, path(i).rgb);
      | end
      | 
      | % show the top name or an X
      | if (exist('ok','var') && ok)
      | 	text(bw*0.5, bh*0.2, tspPath, 'horizontalAlignment', 'center');
      | 	patch(0,0,[1 1 1]);
      | 	patch(bw,bh,[1 1 1]);
      | else
      | 	tx=bw*0.03;
      | 	ty=bh*0.03;
      | 	patch([0 tx bw bw-tx], [ty 0 bh-ty bh], [1 0 0]);
      | 	patch([0 bw-tx bw tx], [bh-ty 0 ty bh], [1 0 0]);
      | end

== system Model_InterpretationEngine64/ModelPreAmp/DecRate/AudioPilot35/Audiopilot_3_5/ConfigurationRtcInputs/APHvac ==
  StateVar : StateVar/StateVar  TriggerInit=[490 139 605 201]  StateName=HvacDbspl
      settings: SourceProductName=Bose Talaria
  TSP : TSP/TSP  TriggerInit=[110 134 215 206]  TspName=HvacDbspl  IfDefMacro=IfdefMacro  Role=Automatic
      settings: SourceProductName=Bose Talaria
  TrivialInterpretation : StateVar/TrivialInterpretation  TriggerInit=[330 148 380 192]
      settings: SourceProductName=Bose Talaria
  wires:
  TSP/1 -> TrivialInterpretation/1
  TrivialInterpretation/1 -> StateVar/1

== system Model_InterpretationEngine64/ModelPreAmp/DecRate/AudioPilot35/Audiopilot_3_5/ConfigurationRtcInputs/VehicleSpeed ==
  StateVar : StateVar/StateVar  TriggerInit=[490 139 605 201]  StateName=VehicleSpeed
      settings: SourceProductName=Bose Talaria
  TSP : TSP/TSP  TriggerInit=[110 134 215 206]  TspName=VehicleSpeed  IfDefMacro=IfdefMacro  Role=Automatic
      settings: SourceProductName=Bose Talaria
  TrivialInterpretation : StateVar/TrivialInterpretation  TriggerInit=[330 148 380 192]
      settings: SourceProductName=Bose Talaria
  wires:
  TSP/1 -> TrivialInterpretation/1
  TrivialInterpretation/1 -> StateVar/1
